simulink model "SlidingModeControl_Example"  (R2019a)
settings: Solver=VariableStepAuto  StartTime=0.0  StopTime=10.0  RelTol=1e-3
settings Model: Creator=0629w  LastModifiedBy=0629w

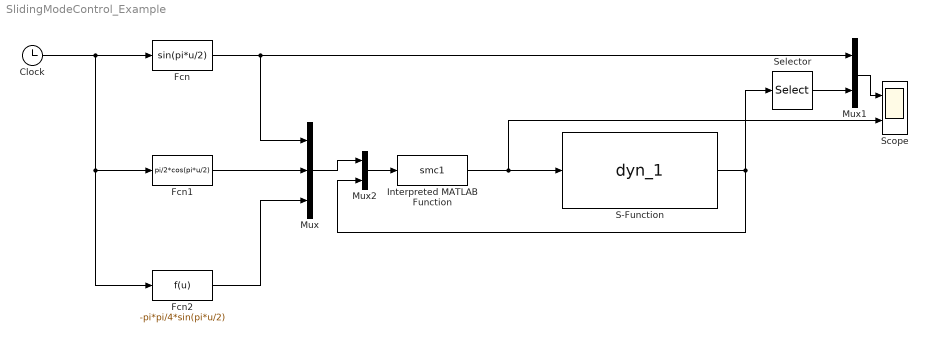
== system SlidingModeControl_Example ==
  Clock : Clock
  Fcn : Fcn  Expr=sin(pi*u/2)
  Fcn1 : Fcn  Expr=pi/2*cos(pi*u/2)
  Fcn2 : Fcn  Expr=-pi*pi/4*sin(pi*u/2)
  Interpreted MATLAB Function : MATLABFcn  MATLABFcn=smc1
  Mux : Mux  Inputs=3
  Mux1 : Mux  Inputs=2
  Mux2 : Mux  Inputs=2
  S-Function : S-Function  FunctionName=dyn_1  SFunctionDeploymentMode=off  EnableBusSupport=off
  Scope : Scope  NumInputPorts=2
  Selector : Selector  InputPortWidth=2  IndexOptions=Index vector (dialog)  Indices=[1]  OutputSizes=1
  wires:
  Fcn/1 -> Mux/1, Mux1/1
  Fcn1/1 -> Mux/2
  Fcn2/1 -> Mux/3
  Clock/1 -> Fcn2/1, Fcn1/1, Fcn/1
  Interpreted MATLAB Function/1 -> Scope/2, S-Function/1
  S-Function/1 -> Mux2/2, Selector/1
  Mux1/1 -> Scope/1
  Selector/1 -> Mux1/2
  Mux/1 -> Mux2/1
  Mux2/1 -> Interpreted MATLAB Function/1
